simulink model "testDynamicVolumetricEfficiency"  (R2023a)
settings: Solver=VariableStepAuto  StartTime=0.0  StopTime=10.0  RelTol=1e-3
libraries: simulink x2
settings Model: Creator=rafael  LastModifiedBy=rafael

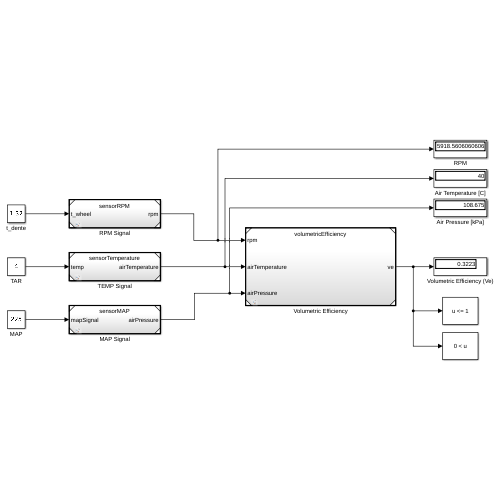
[thumbnail: Simulink's stored preview of the top-level diagram]
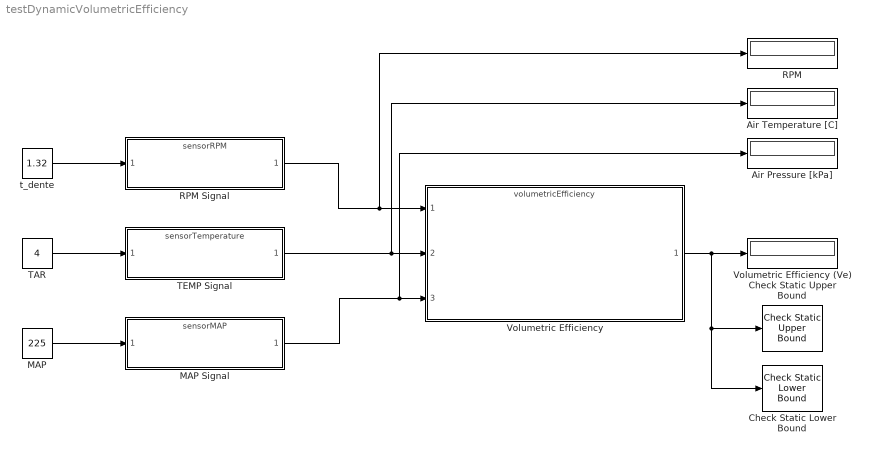
== system testDynamicVolumetricEfficiency ==
  Air Pressure [kPa] : Display
      settings: Format=decimal (Stored Integer)
  Air Temperature [C] : Display
      settings: Format=decimal (Stored Integer)
  Check Static Lower Bound : simulink/Model Verification/Check Static  Lower Bound  Description=0 < u  min=0  min_included=off  enabled=on  stopWhenAssertionFail=on  export=off  icon=text
  Check Static Upper Bound : simulink/Model Verification/Check Static  Upper Bound  Description=u <= 1  max=1  max_included=on  enabled=on  stopWhenAssertionFail=on  export=off  icon=text
  MAP : Constant  Value=225
  MAP Signal : ModelReference  ModelNameDialog=sensorMAP.slx  SimulationMode=Normal  ModelReferenceVersion=1.3
  RPM : Display
      settings: Format=decimal (Stored Integer)
  RPM Signal : ModelReference  ModelNameDialog=sensorRPM.slx  SimulationMode=Normal  ModelReferenceVersion=1.1
  TAR : Constant  Value=4
  TEMP Signal : ModelReference  ModelNameDialog=sensorTemperature.slx  SimulationMode=Normal  ModelReferenceVersion=1.4
  Volumetric Efficiency : ModelReference  ModelNameDialog=volumetricEfficiency.slx  SimulationMode=Normal  ModelReferenceVersion=1.16
  Volumetric Efficiency (Ve) : Display
  t_dente : Constant  Value=1.32
  wires:
  Volumetric Efficiency/1 -> Check Static Lower Bound/1, Check Static Upper Bound/1, Volumetric Efficiency (Ve)/1
  t_dente/1 -> RPM Signal/1
  MAP/1 -> MAP Signal/1
  TAR/1 -> TEMP Signal/1
  MAP Signal/1 -> Volumetric Efficiency/3, Air Pressure [kPa]/1
  TEMP Signal/1 -> Air Temperature [C]/1, Volumetric Efficiency/2
  RPM Signal/1 -> RPM/1, Volumetric Efficiency/1
